simulink model "controller0"  (Simulink 7.7)
settings: Solver=ode45  StartTime=0.0  StopTime=2  RelTol=1e-3
undefined symbols (not defined in the file): scheduler
libraries: simulink_extras x1
settings Model: Creator=tarik  LastModifiedBy=ttosun

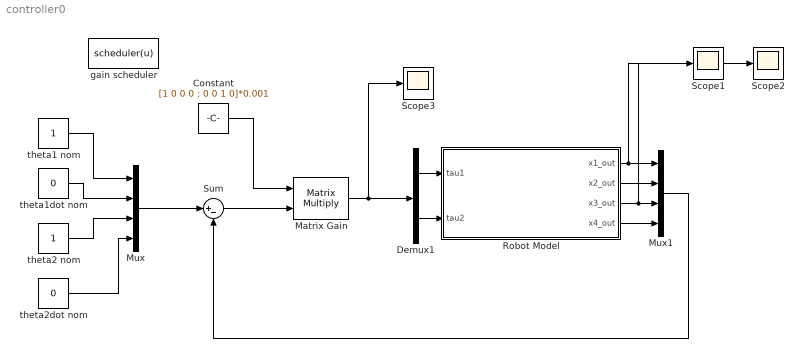
== system controller0 ==
  Constant : Constant  Value=[1 0 0 0 ; 0 0 1 0]*0.001  VectorParams1D=off
  Demux1 : Demux  Outputs=2
  Matrix Gain : Product  Multiplication=Matrix(*)  SampleTime=0.1
  Mux : Mux
  Mux1 : Mux
  Robot Model : Subsystem
  Scope1 : Scope
      settings: YMin=-5e+10  YMax=5e+11
  Scope2 : Scope
      settings: YMin=-5e+10  YMax=5e+11
  Scope3 : Scope
      settings: YMin=-5e+10  YMax=5e+11  SaveName=ScopeData2
  Sum : Sum  Inputs=|+-
  gain scheduler : MATLABFcn  MATLABFcn=scheduler(u)  OutputDimensions=[2,4]  Output1D=off
  theta1 nom : Constant
  theta1dot nom : Constant  Value=0
  theta2 nom : Constant
  theta2dot nom : Constant  Value=0
  wires:
  theta1 nom/1 -> Mux/1
  theta1dot nom/1 -> Mux/2
  theta2 nom/1 -> Mux/3
  theta2dot nom/1 -> Mux/4
  Mux/1 -> Sum/1
  Robot Model/1(x1_out) -> Mux1/1, Scope1/1
  Robot Model/2(x2_out) -> Mux1/2
  Robot Model/3(x3_out) -> Mux1/3, Scope2/1
  Robot Model/4(x4_out) -> Mux1/4
  Mux1/1 -> Sum/2
  Demux1/1 -> Robot Model/1(tau1)
  Demux1/2 -> Robot Model/2(tau2)
  Matrix Gain/1 -> Demux1/1, Scope3/1
  Sum/1 -> Matrix Gain/2
  Constant/1 -> Matrix Gain/1

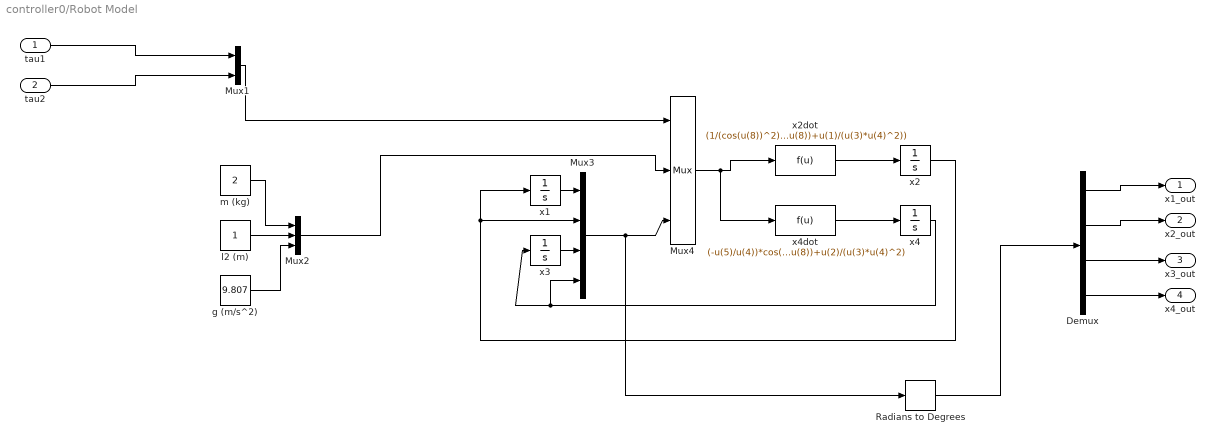
== system controller0/Robot Model ==
  tau1 : Inport
  tau2 : Inport  Port=2
  Demux : Demux
  Mux1 : Mux  Inputs=2
  Mux2 : Mux  Inputs=3
  Mux3 : Mux
  Mux4 : Mux  Description=|  Inputs=3
      | u(1:2) are u1 and u2   
      | u(3:5) are m, l2, and g
      | u(6:9) are x1 x2 x3 x4
  Radians to Degrees : simulink_extras/Transformations/Radians to Degrees  SystemSampleTime=-1
  g (m/s^2) : Constant  Value=9.807
  l2 (m) : Constant
  m (kg) : Constant  Value=2
  x{1..4} (4 alike) : Integrator
  x2dot : Fcn  Expr=(1/(cos(u(8))^2))*(u(7)*u(9)*sin(2*u(8))+u(1)/(u(3)*u(4)^2))
  x4dot : Fcn  Expr=(-u(5)/u(4))*cos(u(8))-(u(7)/2)*sin(2*u(8))+u(2)/(u(3)*u(4)^2)
  x1_out : Outport
  x2_out : Outport  Port=2
  x3_out : Outport  Port=3
  x4_out : Outport  Port=4
  wires:
  m (kg)/1 -> Mux2/1
  l2 (m)/1 -> Mux2/2
  g (m/s^2)/1 -> Mux2/3
  x2dot/1 -> x2/1
  x4dot/1 -> x4/1
  Mux3/1 -> Mux4/3, Radians to Degrees/1
  Mux2/1 -> Mux4/2
  Mux1/1 -> Mux4/1
  x3/1 -> Mux3/3
  x4/1 -> Mux3/4, x3/1
  tau1/1 -> Mux1/1
  tau2/1 -> Mux1/2
  Mux4/1 -> x2dot/1, x4dot/1
  x2/1 -> Mux3/2, x1/1
  x1/1 -> Mux3/1
  Demux/1 -> x1_out/1
  Demux/2 -> x2_out/1
  Demux/3 -> x3_out/1
  Demux/4 -> x4_out/1
  Radians to Degrees/1 -> Demux/1
